simulink model "darko_control_lineaire1"  (R2021b)
settings: Solver=VariableStepAuto  StartTime=0.0  StopTime=12  MaxStep=0.24  RelTol=1e-3
values from neighbouring files (symbols this model uses):
  drone = generateDarko()    [main_linearisation.m]
  initial_state = [p_initial; v_initial; q_initial; omega_initial]    [main_linearisation.m]
  K_complet = [K(:,1:6), zeros(4,1), K(:,7:12)]    [main_linearisation.m]
  S_complet = [S(1:6,1:6), zeros(6,1), S(1:6,7:12); zeros(1,13); S(7:12,1:6), zeros(6,1), S(7:12,7:12)]    [main_linearisation.m]
  u_eq = drone.G*drone.MASS/(2*drone.Fb(1,1)) * [1;1;0;0]    [main_linearisation.m]
  x_eq = [[0; 0; 0]; [0; 0; 0]; eul2quat([yaw, pitch, roll])'; [0; 0; 0]]    [main_linearisation.m]
libraries: simulink_extras x6, sharedtransform x2
settings Model: Creator=florian  LastModifiedBy=florian
settings SolverCC: AlgebraicLoopSolver=TrustRegion
settings DebuggingCC: SFMachineParentedDataDiag=warning

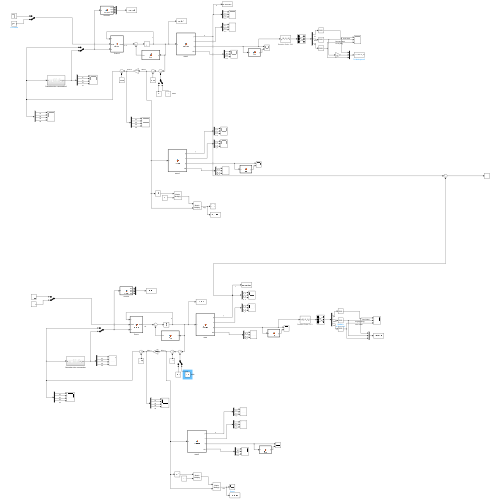
[thumbnail: Simulink's stored preview of the top-level diagram]
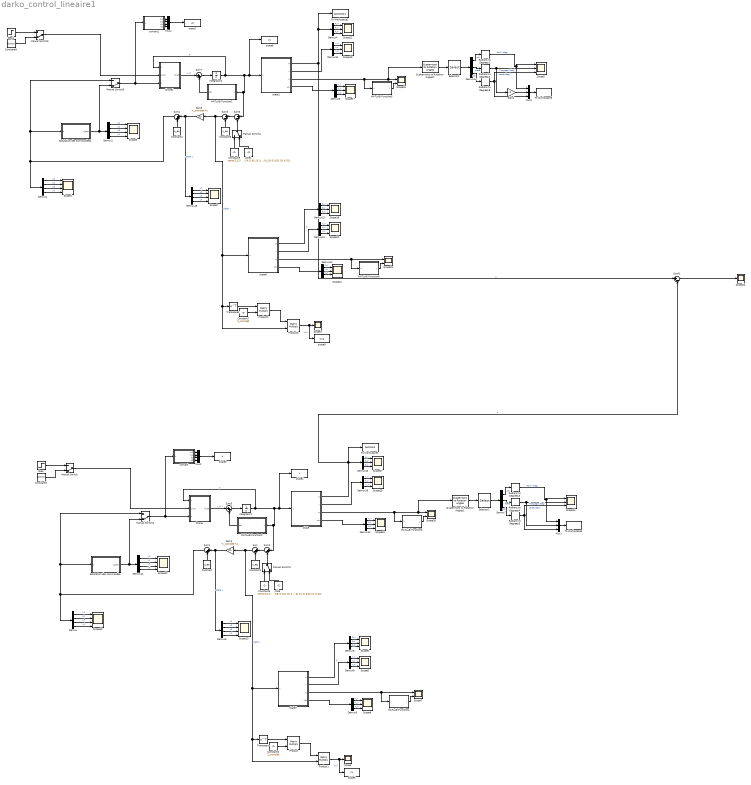
== system darko_control_lineaire1 ==
  Constant : Constant  Value=u_eq
  Constant1 : Constant  Value=x_eq
  Constant2 : Constant  Value=S_complet
  Constant3 : Constant  Value=[0;0;0]
  Constant4 : Constant  Value=u_eq
  Constant5 : Constant  Value=zeros(13,1)
  Constant6 : Constant  Value=x_eq
  Constant7 : Constant  Value=S_complet
  Constant8 : Constant  Value=[0;0;0]
  Constant9 : Constant  Value=zeros(13,1)
  Demux{,1..2,9,11,16} (6 alike) : Demux
  Demux{3..8,10,12..15,24..26} (14 alike) : Demux  Outputs=3
  Drone : MATLAB Function  TreatAsAtomicUnit=on
  Drone1 : MATLAB Function  TreatAsAtomicUnit=on
  Gain1 : Gain  Gain=-K_complet  Multiplication=Matrix(K*u) (u vector)
  Gain3 : Gain  Gain=-K_complet  Multiplication=Matrix(K*u) (u vector)
  Gain4 : Gain  Gain=-1
  Integrator1 : Integrator  InitialCondition=initial_state
  Integrator2 : Integrator  InitialCondition=initial_state
  MATLAB Function1 : MATLAB Function  TreatAsAtomicUnit=on
  MATLAB Function2 : MATLAB Function  TreatAsAtomicUnit=on
  MATLAB Function3 : MATLAB Function  TreatAsAtomicUnit=on
  MATLAB Function4 : MATLAB Function  TreatAsAtomicUnit=on
  MATLAB Function5 : MATLAB Function  TreatAsAtomicUnit=on
  MATLAB Function6 : MATLAB Function  TreatAsAtomicUnit=on
  Manual Switch{,1..5} (6 alike) : ManualSwitch  CurrentSetting=0
  Mux1 : Mux  Inputs=3
  Mux2 : Mux
  Mux3 : Mux  Inputs=3
  Mux4 : Mux
  Product{,1..3} (4 alike) : Product  Multiplication=Matrix(*)
  Quaternions to Rotation Angles1 : sharedtransform/Quaternions to Rotation Angles  rotationOrder=ZXY  aMode=aMode
      settings: SourceProductBaseCode=AE,PW,DR,MT,UV,VE
  Quaternions to Rotation Angles2 : sharedtransform/Quaternions to Rotation Angles  rotationOrder=ZXY  aMode=aMode
      settings: SourceProductBaseCode=AE,PW,DR,MT,UV,VE
  Radians to Degrees{1..6} (6 alike) : simulink_extras/Transformations/Radians to Degrees
  Satutation des commandes : Subsystem
  Satutation des commandes1 : Subsystem
  Scope : Scope
  Scope1 : Scope
  Scope{2..4,10,12..13} (6 alike) : Scope  NumInputPorts=4
  Scope{5..6,8..9,11,14,16..18,20..21,27,29,34} (14 alike) : Scope  NumInputPorts=3
  Scope{7,15,19,28} (4 alike) : Scope  NumInputPorts=2
  Scope22 : Scope
  Selector1 : Selector  InputPortWidth=3  IndexOptions=Index vector (dialog)  Indices=[2 3 1]  OutputSizes=1
  Selector2 : Selector  InputPortWidth=3  IndexOptions=Index vector (dialog)  Indices=[2 3 1]  OutputSizes=1
  Step : Step  Time=10  Before=[0;0;0]  After=[-5;0;0]  SampleTime=0
  Step1 : Step  Time=10  Before=[0;0;0]  After=[-5;0;0]  SampleTime=0
  Sum{,2..3,6,8} (5 alike) : Sum  Inputs=|+-
  Sum{1,4..5,7} (4 alike) : Sum  Inputs=|++
  To Workspace1 : ToWorkspace  VariableName=positions  SampleTime=-1
  To Workspace2 : ToWorkspace  VariableName=positions1  SampleTime=-1
  To Workspace3 : ToWorkspace  VariableName=orientation_deg1  SampleTime=-1
  To Workspace5 : ToWorkspace  VariableName=orientation_deg  SampleTime=-1
  Transpose : Math  Operator=transpose  SaturateOnIntegerOverflow=on
  Transpose1 : Math  Operator=transpose  SaturateOnIntegerOverflow=on
  cible : Constant  Value=[[8; 9; 10]; [0; 0; 0]; [0; 0; 0;0]; [0; 0; 0]];
  cible1 : Constant  Value=[[4; 5; 6]; [0; 0; 0]; [0; 0; 0;0]; [0; 0; 0]];
  convert : MATLAB Function  TreatAsAtomicUnit=on
  convert1 : MATLAB Function  TreatAsAtomicUnit=on
  state : MATLAB Function  TreatAsAtomicUnit=on
  state1 : MATLAB Function  TreatAsAtomicUnit=on
  state2 : MATLAB Function  TreatAsAtomicUnit=on
  state3 : ToWorkspace  VariableName=u  SampleTime=-1
  state4 : ToWorkspace  VariableName=x  SampleTime=-1
  state5 : ToWorkspace  VariableName=Vx  SampleTime=-1
  state6 : MATLAB Function  TreatAsAtomicUnit=on
  state7 : ToWorkspace  VariableName=u1  SampleTime=-1
  state8 : ToWorkspace  VariableName=x1  SampleTime=-1
  state9 : ToWorkspace  VariableName=Vx1  SampleTime=-1
  wires:
  Sum5/1 -> Integrator1/1
  MATLAB Function2/1(cor) -> Sum5/2
  Drone/1(dxdt) -> Sum5/1  "x_d"
  Integrator1/1 -> Drone/1(x), state4/1, state/1(x), Sum2/1, MATLAB Function2/1(x)  "p"
  Demux25/3 -> Scope27/3  "p_z"
  Demux26/2 -> Scope29/2  "v_y"
  Demux24/1 -> Scope34/1  "w_x"
  MATLAB Function3/1(y) -> Scope28/2
  state/3(q) -> MATLAB Function3/1(u), Quaternions to Rotation Angles1/1, Scope28/1
  Demux25/1 -> Scope27/1  "p_x"
  state/4(wb) -> Demux24/1
  Demux24/2 -> Scope34/2  "w_y"
  Demux24/3 -> Scope34/3  "w_z"
  state/2(v) -> Demux26/1
  Demux25/2 -> Scope27/2  "p_y"
  Demux26/3 -> Scope29/3  "v_z"
  Demux26/1 -> Scope29/1  "v_x"
  Gain1/1 -> Demux9/1, Sum1/1  "delta u"
  Constant/1 -> Sum1/2
  Constant1/1 -> Sum/2
  Demux6/3 -> Scope6/3  "p_z"
  Demux8/2 -> Scope8/2  "v_y"
  state2/3(q) -> MATLAB Function4/1(u), Scope7/1
  state2/4(wb) -> Demux5/1
  MATLAB Function4/1(y) -> Scope7/2
  Demux5/2 -> Scope9/2  "w_y"
  Demux8/3 -> Scope8/3  "v_z"
  Demux6/1 -> Scope6/1  "p_x"
  Demux5/1 -> Scope9/1  "w_x"
  Demux8/1 -> Scope8/1  "v_x"
  state2/1(p) -> Demux6/1  "p"
  Demux6/2 -> Scope6/2  "p_y"
  Demux5/3 -> Scope9/3  "w_z"
  state2/2(v) -> Demux8/1
  Demux9/3 -> Scope10/3  "u3"
  Demux9/4 -> Scope10/4  "u4"
  Demux9/1 -> Scope10/1  "u1"
  Demux9/2 -> Scope10/2  "u2"
  Product1/1 -> state5/1, Scope/1  "V(x)"
  Transpose/1 -> Product/1
  Constant2/1 -> Product/2
  Product/1 -> Product1/1
  Manual Switch/1 -> Drone/2(wind)
  Step/1 -> Manual Switch/1
  Constant3/1 -> Manual Switch/2
  cible/1 -> Manual Switch1/2
  Manual Switch1/1 -> Sum2/2
  Constant5/1 -> Manual Switch1/1
  Sum2/1 -> Sum/1
  Demux/1 -> Scope13/1  "u1"
  Demux11/2 -> Scope12/2  "u2"
  Demux11/4 -> Scope12/4  "u4"
  Demux/2 -> Scope13/2  "u2"
  Demux/4 -> Scope13/4  "u4"
  Demux11/1 -> Scope12/1  "u1"
  Demux/3 -> Scope13/3  "u3"
  Sum1/1 -> Satutation des commandes/1(U), Manual Switch2/1, Demux/1
  Satutation des commandes/1(U_sat) -> Manual Switch2/2, Demux11/1
  Demux11/3 -> Scope12/3  "u3"
  Manual Switch2/1 -> Drone/3(u), convert/1(u)
  Sum/1 -> Product1/2, Transpose/1, state2/1(x), Gain1/1  "delta x"
  Demux7/2 -> Radians to Degrees4/1  "theta"
  Radians to Degrees4/1 -> Mux1/2, Scope14/2  "Tangage (deg)"
  Mux1/1 -> To Workspace5/1
  Radians to Degrees5/1 -> Mux1/3, Scope14/3  "Lacet (deg)"
  Quaternions to Rotation Angles1/1 -> Selector1/1
  Demux7/3 -> Radians to Degrees5/1  "psi"
  Selector1/1 -> Demux7/1
  Demux7/1 -> Radians to Degrees3/1  "phi"
  Radians to Degrees3/1 -> Mux1/1, Scope14/1  "Rouli (deg)"
  state/1(p) -> Sum8/2, To Workspace1/1, Demux25/1  "p"
  convert/2(w2) -> Mux2/2
  convert/4(d2) -> Mux2/4
  convert/3(d1) -> Mux2/3
  Mux2/1 -> state3/1
  convert/1(w1) -> Mux2/1
  state6/1(p) -> Demux13/1  "p"
  Constant7/1 -> Product2/2
  Demux16/4 -> Scope2/4  "u4"
  Sum4/1 -> Satutation des commandes1/1(U), Manual Switch5/1, Demux1/1
  Demux15/2 -> Scope20/2  "v_y"
  Constant9/1 -> Manual Switch4/1
  Demux1/2 -> Scope4/2  "u2"
  state6/2(v) -> Demux15/1
  Demux14/1 -> Radians to Degrees1/1  "phi"
  Step1/1 -> Manual Switch3/1
  Demux3/2 -> Scope17/2  "w_y"
  Demux15/1 -> Scope20/1  "v_x"
  Demux10/3 -> Scope16/3  "v_z"
  state6/3(q) -> MATLAB Function6/1(u), Scope19/1
  Gain4/1 -> Mux3/2
  Manual Switch5/1 -> Drone1/3(u), convert1/1(u)
  Demux1/1 -> Scope4/1  "u1"
  Demux1/3 -> Scope4/3  "u3"
  Demux10/1 -> Scope16/1  "v_x"
  Demux12/1 -> Scope21/1  "w_x"
  Product3/1 -> state9/1, Scope1/1  "V(x)"
  convert1/3(d1) -> Mux4/3
  Demux10/2 -> Scope16/2  "v_y"
  Selector2/1 -> Demux14/1
  Demux2/3 -> Scope3/3  "u3"
  Demux14/2 -> Radians to Degrees2/1  "theta"
  Radians to Degrees2/1 -> Gain4/1, Scope5/2  "Tangage (deg)"
  Demux14/3 -> Radians to Degrees6/1  "psi"
  Demux2/1 -> Scope3/1  "u1"
  convert1/4(d2) -> Mux4/4
  Quaternions to Rotation Angles2/1 -> Selector2/1
  Manual Switch4/1 -> Sum6/2
  MATLAB Function6/1(y) -> Scope19/2
  state1/4(wb) -> Demux3/1
  Constant6/1 -> Sum3/2
  Demux12/3 -> Scope21/3  "w_z"
  state1/2(v) -> Demux10/1
  MATLAB Function5/1(y) -> Scope15/2
  Manual Switch3/1 -> Drone1/2(wind)
  convert1/2(w2) -> Mux4/2
  MATLAB Function1/1(cor) -> Sum7/2
  Drone1/1(dxdt) -> Sum7/1  "x_d"
  Demux16/1 -> Scope2/1  "u1"
  Product2/1 -> Product3/1
  Demux4/3 -> Scope11/3  "p_z"
  state6/4(wb) -> Demux12/1
  Demux16/3 -> Scope2/3  "u3"
  Demux13/2 -> Scope18/2  "p_y"
  Radians to Degrees1/1 -> Mux3/1, Scope5/1  "Rouli (deg)"
  Demux2/4 -> Scope3/4  "u4"
  Demux4/1 -> Scope11/1  "p_x"
  Satutation des commandes1/1(U_sat) -> Manual Switch5/2, Demux2/1
  Mux4/1 -> state7/1
  convert1/1(w1) -> Mux4/1
  Demux3/3 -> Scope17/3  "w_z"
  Demux4/2 -> Scope11/2  "p_y"
  Sum7/1 -> Integrator2/1
  state1/3(q) -> MATLAB Function5/1(u), Quaternions to Rotation Angles2/1, Scope15/1
  Demux16/2 -> Scope2/2  "u2"
  Demux13/1 -> Scope18/1  "p_x"
  Demux1/4 -> Scope4/4  "u4"
  Sum6/1 -> Sum3/1
  Constant8/1 -> Manual Switch3/2
  Demux3/1 -> Scope17/1  "w_x"
  Demux13/3 -> Scope18/3  "p_z"
  Demux2/2 -> Scope3/2  "u2"
  state1/1(p) -> Sum8/1, To Workspace2/1, Demux4/1  "p"
  Gain3/1 -> Demux16/1, Sum4/1  "delta u"
  Demux15/3 -> Scope20/3  "v_z"
  Radians to Degrees6/1 -> Mux3/3, Scope5/3  "Lacet (deg)"
  Constant4/1 -> Sum4/2
  Mux3/1 -> To Workspace3/1
  Transpose1/1 -> Product2/1
  cible1/1 -> Manual Switch4/2
  Demux12/2 -> Scope21/2  "w_y"
  Sum3/1 -> Product3/2, Transpose1/1, state6/1(x), Gain3/1  "delta x"
  Integrator2/1 -> Drone1/1(x), state8/1, state1/1(x), Sum6/1, MATLAB Function1/1(x)  "p"
  Sum8/1 -> Scope22/1

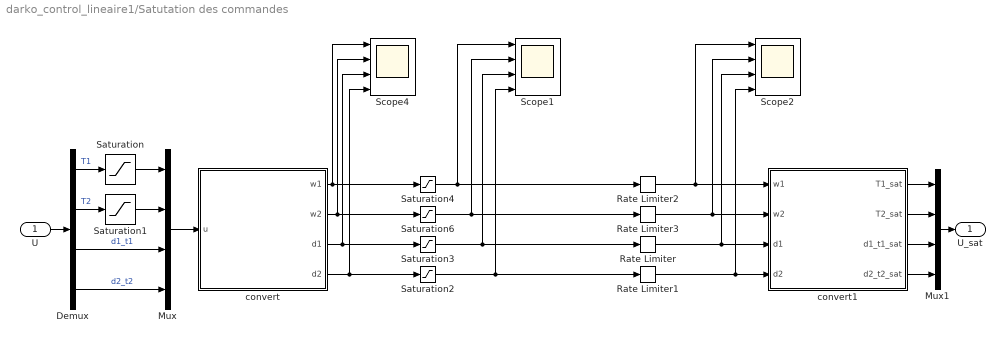
== system darko_control_lineaire1/Satutation des commandes ==
  U : Inport
  Demux : Demux
  Mux : Mux
  Mux1 : Mux
  Rate Limiter : RateLimiter  RisingSlewLimit=drone.ELEVON_RATE_CHANGE  FallingSlewLimit=-drone.ELEVON_RATE_CHANGE  SampleTimeMode=inherited
  Rate Limiter1 : RateLimiter  RisingSlewLimit=drone.ELEVON_RATE_CHANGE  FallingSlewLimit=-drone.ELEVON_RATE_CHANGE  SampleTimeMode=inherited
  Rate Limiter2 : RateLimiter  RisingSlewLimit=drone.MOTOR_RATE_CHANGE  FallingSlewLimit=-drone.MOTOR_RATE_CHANGE  SampleTimeMode=inherited
  Rate Limiter3 : RateLimiter  RisingSlewLimit=drone.MOTOR_RATE_CHANGE  FallingSlewLimit=-drone.MOTOR_RATE_CHANGE  SampleTimeMode=inherited
  Saturation : Saturate  UpperLimit=100  LowerLimit=0.001
  Saturation1 : Saturate  UpperLimit=100  LowerLimit=0.001
  Saturation2 : Saturate  UpperLimit=30*(pi/180)  LowerLimit=-30*(pi/180)
  Saturation3 : Saturate  UpperLimit=30*(pi/180)  LowerLimit=-30*(pi/180)
  Saturation4 : Saturate  UpperLimit=1000  LowerLimit=200
  Saturation6 : Saturate  UpperLimit=1000  LowerLimit=200
  Scope1 : Scope  NumInputPorts=4
  Scope2 : Scope  NumInputPorts=4
  Scope4 : Scope  NumInputPorts=4
  convert : MATLAB Function  TreatAsAtomicUnit=on
  convert1 : MATLAB Function  TreatAsAtomicUnit=on
  U_sat : Outport
  wires:
  U/1 -> Demux/1
  Demux/4 -> Mux/4  "d2_t2"
  Demux/1 -> Saturation/1  "T1"
  Demux/3 -> Mux/3  "d1_t1"
  Demux/2 -> Saturation1/1  "T2"
  Saturation/1 -> Mux/1
  Mux/1 -> convert/1(u)
  convert/1(w1) -> Saturation4/1, Scope4/1
  Saturation3/1 -> Rate Limiter/1, Scope1/3
  convert/2(w2) -> Scope4/2, Saturation6/1
  convert/3(d1) -> Scope4/3, Saturation3/1
  convert/4(d2) -> Saturation2/1, Scope4/4
  convert1/1(T1_sat) -> Mux1/1
  convert1/4(d2_t2_sat) -> Mux1/4
  Mux1/1 -> U_sat/1
  Saturation1/1 -> Mux/2
  convert1/2(T2_sat) -> Mux1/2
  convert1/3(d1_t1_sat) -> Mux1/3
  Saturation2/1 -> Rate Limiter1/1, Scope1/4
  Rate Limiter/1 -> Scope2/3, convert1/3(d1)
  Saturation6/1 -> Rate Limiter3/1, Scope1/2
  Saturation4/1 -> Rate Limiter2/1, Scope1/1
  Rate Limiter1/1 -> Scope2/4, convert1/4(d2)
  Rate Limiter2/1 -> Scope2/1, convert1/1(w1)
  Rate Limiter3/1 -> Scope2/2, convert1/2(w2)

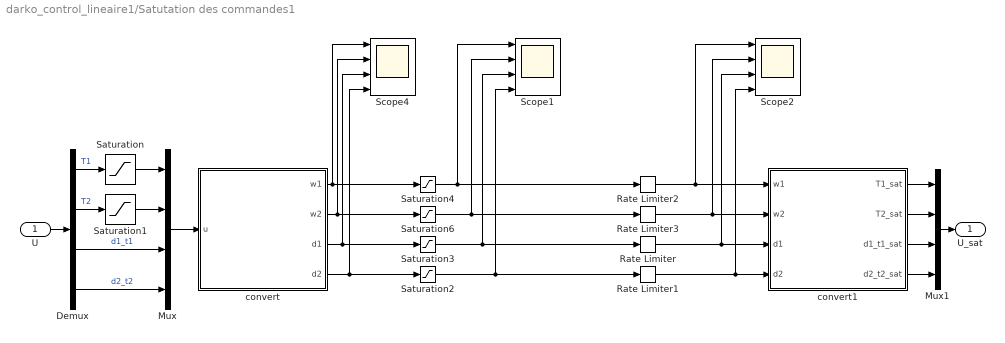
== system darko_control_lineaire1/Satutation des commandes1 ==
  U : Inport
  Demux : Demux
  Mux : Mux
  Mux1 : Mux
  Rate Limiter : RateLimiter  RisingSlewLimit=drone.ELEVON_RATE_CHANGE  FallingSlewLimit=-drone.ELEVON_RATE_CHANGE  SampleTimeMode=inherited
  Rate Limiter1 : RateLimiter  RisingSlewLimit=drone.ELEVON_RATE_CHANGE  FallingSlewLimit=-drone.ELEVON_RATE_CHANGE  SampleTimeMode=inherited
  Rate Limiter2 : RateLimiter  RisingSlewLimit=drone.MOTOR_RATE_CHANGE  FallingSlewLimit=-drone.MOTOR_RATE_CHANGE  SampleTimeMode=inherited
  Rate Limiter3 : RateLimiter  RisingSlewLimit=drone.MOTOR_RATE_CHANGE  FallingSlewLimit=-drone.MOTOR_RATE_CHANGE  SampleTimeMode=inherited
  Saturation : Saturate  UpperLimit=100  LowerLimit=0.001
  Saturation1 : Saturate  UpperLimit=100  LowerLimit=0.001
  Saturation2 : Saturate  UpperLimit=30*(pi/180)  LowerLimit=-30*(pi/180)
  Saturation3 : Saturate  UpperLimit=30*(pi/180)  LowerLimit=-30*(pi/180)
  Saturation4 : Saturate  UpperLimit=1000  LowerLimit=200
  Saturation6 : Saturate  UpperLimit=1000  LowerLimit=200
  Scope1 : Scope  NumInputPorts=4
  Scope2 : Scope  NumInputPorts=4
  Scope4 : Scope  NumInputPorts=4
  convert : MATLAB Function  TreatAsAtomicUnit=on
  convert1 : MATLAB Function  TreatAsAtomicUnit=on
  U_sat : Outport
  wires:
  U/1 -> Demux/1
  Demux/4 -> Mux/4  "d2_t2"
  Demux/1 -> Saturation/1  "T1"
  Demux/3 -> Mux/3  "d1_t1"
  Demux/2 -> Saturation1/1  "T2"
  Saturation/1 -> Mux/1
  Mux/1 -> convert/1(u)
  convert/1(w1) -> Saturation4/1, Scope4/1
  Saturation3/1 -> Rate Limiter/1, Scope1/3
  convert/2(w2) -> Scope4/2, Saturation6/1
  convert/3(d1) -> Scope4/3, Saturation3/1
  convert/4(d2) -> Saturation2/1, Scope4/4
  convert1/1(T1_sat) -> Mux1/1
  convert1/4(d2_t2_sat) -> Mux1/4
  Mux1/1 -> U_sat/1
  Saturation1/1 -> Mux/2
  convert1/2(T2_sat) -> Mux1/2
  convert1/3(d1_t1_sat) -> Mux1/3
  Saturation2/1 -> Rate Limiter1/1, Scope1/4
  Rate Limiter/1 -> Scope2/3, convert1/3(d1)
  Saturation6/1 -> Rate Limiter3/1, Scope1/2
  Saturation4/1 -> Rate Limiter2/1, Scope1/1
  Rate Limiter1/1 -> Scope2/4, convert1/4(d2)
  Rate Limiter2/1 -> Scope2/1, convert1/1(w1)
  Rate Limiter3/1 -> Scope2/2, convert1/2(w2)

== matlab function darko_control_lineaire1/convert1 ==
  data: u input; w1 output; drone parameter; w2 output; d1 output; d2 output
function [w1, w2, d1, d2] = convert(u, drone)
%#codegen
kf = drone.PROP_KP;

T1 = max(u(1),0);
T2 = max(u(2),0);
d1_T1 = u(3);
d2_T2 = u(4);

w1 = sqrt(T1/kf)*60/(2*pi);
w2 = sqrt(T2/kf)*60/(2*pi);
d1 = d1_T1/T1 *(360/(2*pi));
d2 = d2_T2/T2*(360/(2*pi));

== matlab function darko_control_lineaire1/Satutation des commandes/convert1 ==
  data: w1 input; w2 input; d1 input; d2 input; T1_sat output; T2_sat output; drone parameter; d1_t1_sat output; d2_t2_sat output
function [T1_sat, T2_sat, d1_t1_sat, d2_t2_sat] = convert2(w1, w2, d1, d2, drone)
%#codegen
kf = drone.PROP_KP;

T1_sat = kf*w1^2;
d1_t1_sat = d1*T1_sat;
T2_sat = kf*w2^2;
d2_t2_sat = d2*T2_sat;

== matlab function darko_control_lineaire1/state1 ==
  data: x input; p output; v output; q output; wb output
function [p, v, q, wb] = demux(x)
%#codegen

p = x(1:3);
v = x(4:6);
q  = x(7:10);
wb = x(11:13);

== matlab function darko_control_lineaire1/state6 ==
  data: x input; p output; v output; q output; wb output
function [p, v, q, wb] = demux(x)
%#codegen

p = x(1:3);
v = x(4:6);
q  = x(7:10);
wb = x(11:13);

== matlab function darko_control_lineaire1/Drone1 ==
  data: x input; wind input; u input; dxdt output; drone parameter
function dxdt  = drone(x,wind, u, drone)

%% physical constants
% gravity
g = drone.G;
% vehicle mass
m = drone.MASS;
% vehicle inertia matrix
J = drone.INERTIA; % [3x3 real symmetric] in body axis

%% state demultiplexing
% p = x(1:3);
v = x(4:6);
q  = x(7:10);
wb = x(11:13);

Rq = q2dcm(q);

[Fp, Mp] = external_force_moment(x, u, wind, drone);

% position
dpdt = v;

% kinematics
dvdt =  [0;0;g] + (1/m)*Rq*drone.Fb*u; %+ (1/m)*Rq*Fp; 

%% quaternion derivative
eta = q(1);
eps = q(2:4);

dqdt = (1/2)*[-eps'; eta*eye(3) + skew_sym(eps)]*wb;

%% angular velocity derivative
% kinematics
dwdt = -J\cross(wb, J*wb) + J\(drone.Mb*u);% + J\Mp;


%% derivative multiplexing
dxdt = [dpdt; dvdt; dqdt; dwdt] ;

== matlab function darko_control_lineaire1/MATLAB Function2 ==
  data: x input; cor output
function cor  = fcn(x)
%#codegen
q  = x(7:10);
n = norm(q);
mismatch = 1-n;
cor = [0;0;0; 0;0;0; mismatch*q; 0;0;0];

== matlab function darko_control_lineaire1/MATLAB Function3 ==
  data: u input; y output
function y = fcn(u)
%#codegen

y = norm(u);

== matlab function darko_control_lineaire1/convert ==
  data: u input; w1 output; drone parameter; w2 output; d1 output; d2 output
function [w1, w2, d1, d2] = convert(u, drone)
%#codegen
kf = drone.PROP_KP;

T1 = max(u(1),0);
T2 = max(u(2),0);
d1_T1 = u(3);
d2_T2 = u(4);

w1 = sqrt(T1/kf)*60/(2*pi);
w2 = sqrt(T2/kf)*60/(2*pi);
d1 = d1_T1/T1 *(360/(2*pi));
d2 = d2_T2/T2*(360/(2*pi));

== matlab function darko_control_lineaire1/state ==
  data: x input; p output; v output; q output; wb output
function [p, v, q, wb] = demux(x)
%#codegen

p = x(1:3);
v = x(4:6);
q  = x(7:10);
wb = x(11:13);

== matlab function darko_control_lineaire1/Drone ==
  data: x input; wind input; u input; dxdt output; drone parameter
function dxdt  = drone(x,wind, u, drone)

%% physical constants
% gravity
g = drone.G;
% vehicle mass
m = drone.MASS;
% vehicle inertia matrix
J = drone.INERTIA; % [3x3 real symmetric] in body axis

%% state demultiplexing
% p = x(1:3);
v = x(4:6);
q  = x(7:10);
wb = x(11:13);

Rq = q2dcm(q);

[Fp, Mp] = external_force_moment(x, u, wind, drone);

% position
dpdt = v;

% kinematics
dvdt =  [0;0;g] + (1/m)*Rq*drone.Fb*u + (1/m)*Rq*Fp; 

%% quaternion derivative
eta = q(1);
eps = q(2:4);

dqdt = (1/2)*[-eps'; eta*eye(3) + skew_sym(eps)]*wb;

%% angular velocity derivative
% kinematics
dwdt = -J\cross(wb, J*wb) + J\(drone.Mb*u) + J\Mp;


%% derivative multiplexing
dxdt = [dpdt; dvdt; dqdt; dwdt] ;

== matlab function darko_control_lineaire1/MATLAB Function1 ==
  data: x input; cor output
function cor  = fcn(x)
%#codegen
q  = x(7:10);
n = norm(q);
mismatch = 1-n;
cor = [0;0;0; 0;0;0; mismatch*q; 0;0;0];

== matlab function darko_control_lineaire1/MATLAB Function4 ==
  data: u input; y output
function y = fcn(u)
%#codegen

y = norm(u);

== matlab function darko_control_lineaire1/state2 ==
  data: x input; p output; v output; q output; wb output
function [p, v, q, wb] = demux(x)
%#codegen

p = x(1:3);
v = x(4:6);
q  = x(7:10);
wb = x(11:13);

== matlab function darko_control_lineaire1/MATLAB Function5 ==
  data: u input; y output
function y = fcn(u)
%#codegen

y = norm(u);

== matlab function darko_control_lineaire1/MATLAB Function6 ==
  data: u input; y output
function y = fcn(u)
%#codegen

y = norm(u);

== matlab function darko_control_lineaire1/Satutation des commandes1/convert ==
  data: u input; w1 output; drone parameter; w2 output; d1 output; d2 output
function [w1, w2, d1, d2] = convert(u, drone)
%#codegen
kf = drone.PROP_KP;

T1 = u(1);
T2 = u(2);
d1_T1 = u(3);
d2_T2 = u(4);

w1 = sqrt(T1/kf);
w2 = sqrt(T2/kf);
d1 = d1_T1/T1;
d2 = d2_T2/T2;

== matlab function darko_control_lineaire1/Satutation des commandes1/convert1 ==
  data: w1 input; w2 input; d1 input; d2 input; T1_sat output; T2_sat output; drone parameter; d1_t1_sat output; d2_t2_sat output
function [T1_sat, T2_sat, d1_t1_sat, d2_t2_sat] = convert2(w1, w2, d1, d2, drone)
%#codegen
kf = drone.PROP_KP;

T1_sat = kf*w1^2;
d1_t1_sat = d1*T1_sat;
T2_sat = kf*w2^2;
d2_t2_sat = d2*T2_sat;

== matlab function darko_control_lineaire1/Satutation des commandes/convert ==
  data: u input; w1 output; drone parameter; w2 output; d1 output; d2 output
function [w1, w2, d1, d2] = convert(u, drone)
%#codegen
kf = drone.PROP_KP;

T1 = u(1);
T2 = u(2);
d1_T1 = u(3);
d2_T2 = u(4);

w1 = sqrt(T1/kf);
w2 = sqrt(T2/kf);
d1 = d1_T1/T1;
d2 = d2_T2/T2;
